simulink model "acoustic_delay_buffer"  (Simulink 9.2)
settings: Solver=FixedStepDiscrete  StartTime=0  StopTime=acoustic_delay_buffer_param.endTime  RelTol=1e-3  EnableMultiTasking=on
PreLoadFcn:
  | % Run the setup script when the model is opened
  | setup_acoustic_delay_buffer;
InitFcn:
  | % Run the setup script again just before the
  | % model is run, so that any updates made
  | % after opening are applied.
  | setup_acoustic_delay_buffer;
undefined symbols (not defined in the file or in its folder): acoustic_delay_buffer_param, AdvDSPBChannelOutDisplay, AdvDSPBDMemDisplay, AStInput, AStOutput, dpoly, dspba_ChannelInVis, dspba_ChannelOutVis, dspba_internal_get_channel_ports, DSPBAAvalonST, evalAionMaskParam, latency, primtype, UseDontCare, value
libraries: DSPBAPrim x45, simulink x4, DSPBABase x3, DSPBAModelBus x2
(part 1 of 2)
Description:
  | DSP Builder Advanced Template for Template Design implementing ModelIP designs
settings Model: LogicAnalyzerSignalOrdering=673dd956-a9b7-47c6-8e3b-b5370a165700,2ca13bd6-3b11-4a64-9ccb-860d4470aa9c,1314958b-2ca4-4760-b14e-21636fc16e8a,18024acf-8c31-4ed4-966b-9c5112f68f18,b16340d5-95cc-41ce-b9ba-3d9f2a82d5c7,73847741-1302-4618-ba98-6acef04c4683,30466ab8-321b-45d2-abc5-98b1f25c16af,0661e296-95ee-4d47-9664-915a724506db,a1263464-d66d-421f-b545-d698760bf497,336fe2d9-f44c-47a9-a8e5-5e40221b217f,f71103e9-4e69-4618-a9ca-5008dd724a19,a742d53d-581d-4b05-b348-192446bdeb24,b655c0ea-e5b7-4f9a-9095-04efa7391f59,5190fdba-c9e1-4656-be28-b079149338cb,ddf50ec1-edd7-49e5-a566-ac4f62c951d6,aaf5a439-c955-4ee6-b568-777acc1bd3bb,ac04c1fb-3b27-4459-9e9c-8231ad8ef4bf,6258e434-ad41-4b37-b0cd-7eb737f716c4,09754ba2-98e9-4803-bde8-10590804ee7c  Creator=mjervis  LastModifiedBy=trevorvannoy
settings Model: SuppressorTable=|
  | <?xml version="1.0" encoding="UTF-8" standalone="yes" ?>
  | <!DOCTYPE boost_serialization>
  | <boost_serialization signature="serialization::archive" version="15">
  | <DiagnosticSuppressor class_id="0" tracking_level="0" version="6">
  | 	<Table class_id="1" tracking_level="0" version="0">
  | 		<count>2</count>
  | 		<bucket_count>8</bucket_count>
  | 		<item_version>0</item_version>
  | 		<item class_id="2" tracking_level="0" version="0">
  | 			<first class_id="3" tracking_level="0" version="6">
  | 				<Source class_id="4" tracking_level="0" version="0">
  | 					<count>1</count>
  | 					<item_version>0</item_version>
  | 					<item>acoustic_delay_buffer/channel/LimitedCounter</item>
  | 				</Source>
  | 			</first>
  | 			<second class_id="5" tracking_level="0" version="6">
  | 				<SuppressedData class_id="6" tracking_level="0" version="0">
  | 					<count>2</count>
  | 					<bucket_count>8</bucket_count>
  | 					<item_version>0</item_version>
  | 					<item class_id="7" tracking_level="0" version="0">
  | 						<first class_id="8" tracking_level="0" version="6">
  | 							<ID>SimulinkFixedPoint:util:Overflowoccurred</ID>
  | 							<Cause>
  | 								<Source>
  | 									<count>0</count>
  | 									<item_version>0</item_version>
  | 								</Source>
  | 							</Cause>
  | 						</first>
  | 						<second class_id="9" tracking_level="0" version="6">
  | 							<Comment></Comment>
  | 							<User></User>
  | 							<LastModified class_id="10" tracking_level="0" version="0">
  | 								<ptime_date class_id="11" tracking_level="0" version="0">
  | 									<date>20160608</date>
  | 								</ptime_date>
  | 								<ptime_time_duration class_id="12" tracking_level="0" version="0">
  | 									<is_special>0</is_special>
  | 									<time_duration_hours>15</time_duration_hours>
  | 									<time_duration_minutes>23</time_duration_minutes>
  | 									<time_duration_seconds>17</time_duration_seconds>
  | 									<time_duration_fractional_seconds>0</time_duration_fractional_seconds>
  | 								</ptime_time_duration>
  | 							</LastModified>
  | 							<SuppressionType>1</SuppressionType>
  | 						</second>
  | 					</item>
  | 					<item>
  | 						<first>
  | 							<ID>Simulink:DataType:WarningOverFlowDetected</ID>
  | 							<Cause>
  | 								<Source>
  | 									<count>0</count>
  | 									<item_version>0</item_version>
  | 								</Source>
  | 							</Cause>
  | 						</first>
  | 						<second>
  | 							<Comment></Comment>
  | 							<User></User>
  | 							<LastModified>
  | 								<ptime_date>
  | 									<date>20160608</date>
  | 								</ptime_date>
  | 								<ptime_time_duration>
  | 									<is_special>0</is_special>
  | 									<time_duration_hours>15</time_duration_hours>
  | 									<time_duration_minutes>23</time_duration_minutes>
  | 									<time_duration_seconds>17</time_duration_seconds>
  | 									<time_duration_fractional_seconds>0</time_duration_fractional_seconds>
  | 								</ptime_time_duration>
  | 							</LastModified>
  | 							<SuppressionType>1</SuppressionType>
  | 						</second>
  | 					</item>
  | 				</SuppressedData>
  | 			</second>
  | 		</item>
  | 		<item>
  | 			<first>
  | 				<Source>
  | 					<count>1</count>
  | 					<item_version>0</item_version>
  | 					<item>acoustic_delay_buffer/adb/delay_write_en/LimitedCounter</item>
  | 				</Source>
  | 			</first>
  | 			<second>
  | 				<SuppressedData>
  | 					<count>2</count>
  | 					<bucket_count>8</bucket_count>
  | 					<item_version>0</item_version>
  | 					<item>
  | 						<first>
  | 							<ID>SimulinkFixedPoint:util:Overflowoccurred</ID>
  | 							<Cause>
  | 								<Source>
  | 									<count>0</count>
  | 									<item_version>0</item_version>
  | 								</Source>
  | 							</Cause>
  | 						</first>
  | 						<second>
  | 							<Comment></Comment>
  | 							<User></User>
  | 							<LastModified>
  | 								<ptime_date>
  | 									<date>20160608</date>
  | 								</ptime_date>
  | 								<ptime_time_duration>
  | 									<is_special>0</is_special>
  | 									<time_duration_hours>15</time_duration_hours>
  | 									<time_duration_minutes>23</time_duration_minutes>
  | 									<time_duration_seconds>17</time_duration_seconds>
  | 									<time_duration_fractional_seconds>0</time_duration_fractional_seconds>
  | 								</ptime_time_duration>
  | 							</LastModified>
  | 							<SuppressionType>1</SuppressionType>
  | 						</second>
  | 					</item>
  | 					<item>
  | 						<first>
  | 							<ID>Simulink:DataType:WarningOverFlowDetected</ID>
  | 							<Cause>
  | 								<Source>
  | 									<count>0</count>
  | 									<item_version>0</item_version>
  | 								</Source>
  | 							</Cause>
  | 						</first>
  | 						<second>
  | 							<Comment></Comment>
  | 							<User></User>
  | 							<LastModified>
  | 								<ptime_date>
  | 									<date>20160608</date>
  | 								</ptime_date>
  | 								<ptime_time_duration>
  | 									<is_special>0</is_special>
  | 									<time_duration_hours>15</time_duration_hours>
  | 									<time_duration_minutes>23</time_duration_minutes>
  | 									<time_duration_seconds>17</time_duration_seconds>
  | 									<time_duration_fractional_seconds>0</time_duration_fractional_seconds>
  | 								</ptime_time_duration>
  | 							</LastModified>
  | 							<SuppressionType>1</SuppressionType>
  | 						</second>
  | 					</item>
  | 				</SuppressedData>
  | 			</second>
  | 		</item>
  | 	</Table>
  | </DiagnosticSuppressor>
  | </boost_serialization>
settings Model: LogicAnalyzerGraphicalSettings=|
  | {
  |   "cursors" : {
  |     "activeCursor" : 0,
  |     "lockedCursors" : [
  | 
  |     ],
  |     "startingCursor" : 0,
  |     "times" : [
  |       1382
  |     ]
  |   },
  |   "global" : {
  |     "booleanDisplay" : "gradient",
  |     "color" : "#0073bd",
  |     "displayBusElementNames" : true,
  |     "displayShortNames" : true,
  |     "fontSize" : 12,
  |     "height" : 20,
  |     "recentlyUsedColors" : [
  |       "#7d2e8f",
  |       "#0073bd",
  |       "#0fffff",
  |       "default",
  |       "",
  |       "#ffff11",
  |       "#139fff"
  |     ]
  |   },
  |   "panels" : [
  |     {
  |       "height" : 100,
  |       "startingTrace" : 0,
  |       "traces" : [
  |         {
  |           "color" : "#ff6929",
  |           "height" : 30,
  |           "name" : "valid_stim",
  |           "signalId" : "18024acf-8c31-4ed4-966b-9c5112f68f18",
  |           "type" : "wave"
  |         },
  |         {
  |           "color" : "#ff6929",
  |           "height" : 30,
  |           "name" : "channel_stim",
  |           "signalId" : "b16340d5-95cc-41ce-b9ba-3d9f2a82d5c7",
  |           "type" : "wave"
  |         },
  |         {
  |           "color" : "#ff6929",
  |           "height" : 30,
  |           "name" : "data_stim",
  |           "signalId" : "73847741-1302-4618-ba98-6acef04c4683",
  |           "type" : "wave"
  |         },
  |         {
  |           "color" : "#0073bd",
  |           "height" : 30,
  |           "signalId" : "aaf5a439-c955-4ee6-b568-777acc1bd3bb",
  |           "type" : "wave"
  |         },
  |         {
  |           "color" : "#0073bd",
  |           "height" : 30,
  |           "signalId" : "ac04c1fb-3b27-4459-9e9c-8231ad8ef4bf",
  |           "type" : "wave"
  |         },
  |         {
  |           "color" : "#0073bd",
  |           "height" : 30,
  |           "signalId" : "ddf50ec1-edd7-49e5-a566-ac4f62c951d6",
  |           "type" : "wave"
  |         },
  |         {
  |           "color" : "#edb021",
  |           "height" : 30,
  |           "name" : "write_addr == delay",
  |           "signalId" : "1314958b-2ca4-4760-b14e-21636fc16e8a",
  |           "type" : "wave"
  |         },
  |         {
  |           "color" : "#edb021",
  |           "height" : 30,
  |           "name" : "valid_in",
  |           "signalId" : "a1263464-d66d-421f-b545-d698760bf497",
  |           "type" : "wave"
  |         },
  |         {
  |           "color" : "#b746ff",
  |           "height" : 30,
  |           "name" : "din",
  |           "signalId" : "336fe2d9-f44c-47a9-a8e5-5e40221b217f",
  |           "type" : "wave"
  |         },
  |         {
  |           "color" : "#b746ff",
  |           "height" : 30,
  |           "name" : "write",
  |           "signalId" : "a742d53d-581d-4b05-b348-192446bdeb24",
  |           "type" : "wave"
  |         },
  |         {
  |           "color" : "#b746ff",
  |           "height" : 30,
  |           "name" : "write_addr",
  |           "signalId" : "f71103e9-4e69-4618-a9ca-5008dd724a19",
  |           "type" : "wave"
  |         },
  |         {
  |           "color" : "#b746ff",
  |           "height" : 30,
  |           "name" : "read_addr",
  |           "signalId" : "b655c0ea-e5b7-4f9a-9095-04efa7391f59",
  |           "type" : "wave"
  |         },
  |         {
  |           "color" : "#b746ff",
  |           "height" : 30,
  |           "name" : "q1",
  |           "signalId" : "6258e434-ad41-4b37-b0cd-7eb737f716c4",
  |           "type" : "wave"
  |         },
  |         {
  |           "color" : "#b746ff",
  |           "height" : 30,
  |           "name" : "q2",
  |           "signalId" : "09754ba2-98e9-4803-bde8-10590804ee7c",
  |           "type" : "wave"
  |         },
  |         {
  |           "color" : "#78ab30",
  |           "height" : 30,
  |           "name" : "dout_buffer",
  |           "signalId" : "5190fdba-c9e1-4656-be28-b079149338cb",
  |           "type" : "wave"
  |         },
  |         {
  |           "color" : "#78ab30",
  |           "height" : 30,
  |           "name" : "ch_out_buffer",
  |           "signalId" : "30466ab8-321b-45d2-abc5-98b1f25c16af",
  |           "type" : "wave"
  |         },
  |         {
  |           "color" : "#78ab30",
  |           "height" : 30,
  |           "name" : "valid_out_buffer",
  |           "signalId" : "0661e296-95ee-4d47-9664-915a724506db",
  |           "type" : "wave"
  |         },
  |         {
  |           "color" : "#ff13a6",
  |           "height" : 30,
  |           "name" : "reset",
  |           "signalId" : "2ca13bd6-3b11-4a64-9ccb-860d4470aa9c",
  |           "type" : "wave"
  |         },
  |         {
  |           "color" : "#ff13a6",
  |           "height" : 30,
  |           "name" : "delay_comp",
  |           "signalId" : "673dd956-a9b7-47c6-8e3b-b5370a165700",
  |           "type" : "wave"
  |         }
  |       ],
  |       "yOffset" : 0
  |     }
  |   ],
  |   "timeAxis" : {
  |     "pixelsPerSecond" : 0.2014684101347109
  |   },
  |   "trigger" : {
  |     "enabled" : false,
  |     "mode" : "once",
  |     "samples" : 200,
  |     "signals" : {
  |     },
  |     "stages" : [
  |       {
  |         "conditions" : [
  | 
  |         ],
  |         "operator" : "AND"
  |       }
  |     ]
  |   }
  | }
settings DataIOCC: SignalLoggingSaveFormat=Dataset
settings OptimizationCC: BlockReduction=off  ConditionallyExecuteInputs=off  ExpressionDepthLimit=2147483647
settings DebuggingCC: SolverPrmCheckMsg=warning  InheritedTsInSrcMsg=none  MultiTaskRateTransMsg=warning  IntegerOverflowMsg=none  IntegerSaturationMsg=none

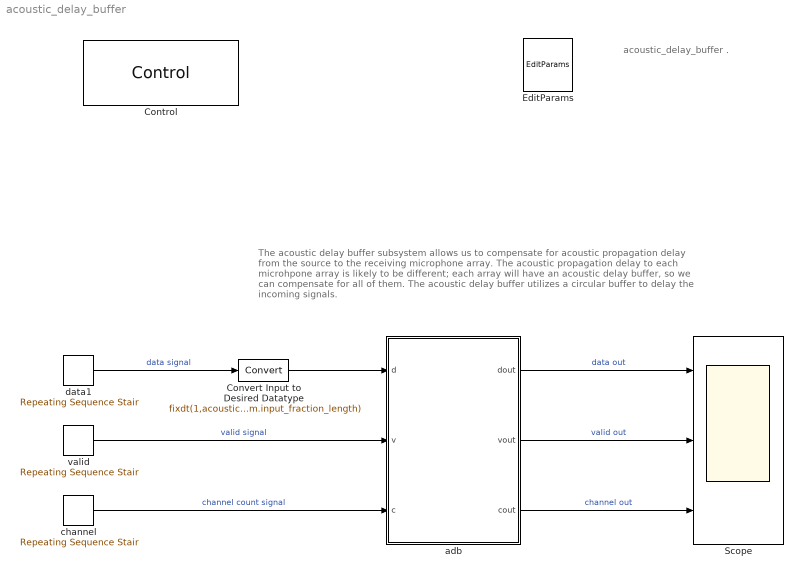
== system acoustic_delay_buffer ==
  note: The acoustic delay buffer subsystem allows us to compensate for acoustic propagation delay from the source to the receiving microphone array. The acoustic propagation delay to each microhpone array is likely to be different; each array will have an acoustic delay buffer, so we can compensate for all of them.
      |
      | The acoustic delay buffer utilizes a circular buffer to delay the incoming signals.
  note: acoustic_delay_buffer
      |                                          .
  Control : DSPBABase/Control  generate=on  language=VHDL  destination=./rtl  destination_gui=./rtl  make_full_path=off  quartus_work=../rtl  quartus_work_gui=../rtl  path_is_relative=on  autotestbench=off  signaldepth=2  coveragetestbench=off  logs=off  spacewidth=2  spacenum=1  addrwidth=10  datawidth=16  dataendian=Big Endian  hierarchicalnames=off  ramThresholdBits=-1  distRamThresholdBits=-1  mlabThresholdBits=-1  hardMultiplierThresholdLuts=-1  version=20090407  errorOnChanMismatch=on  errorOnGPIOMismatch=off  importModelsimResults=0  floatMismatchTolerance=-1.0  floatMismatchZeroTolerance=-1.0  cycleAccurate=off  reinterpretCastMult=off  paramFile=acoustic_delay_buffer_params.xml
  Convert Input to Desired Datatype : DataTypeConversion  OutDataTypeStr=fixdt(1,acoustic_delay_buffer_param.input_word_length,acoustic_delay_buffer_param.input_fraction_length)  SaturateOnIntegerOverflow=on
  EditParams : DSPBABase/EditParams  version=20090407
  Scope : Scope  NumInputPorts=3
  adb : Subsystem  TreatAsAtomicUnit=on
  channel : simulink/Sources/Repeating Sequence Stair  OutValues=acoustic_delay_buffer_param.chan_stim  tsamp=acoustic_delay_buffer_param.ClockCycle  OutMin=[]  OutMax=[]  OutDataTypeStr=uint8  OutputDataTypeScalingMode=uint8  OutDataType=uint8  ConRadixGroup=Best Precision: Vector-wise  OutScaling=2^-12
  data1 : simulink/Sources/Repeating Sequence Stair  OutValues=acoustic_delay_buffer_param.input_data  tsamp=acoustic_delay_buffer_param.ClockCycle  OutMin=[]  OutMax=[]  OutDataTypeStr=Inherit: Inherit via back propagation  OutDataType=fixdt('sfix16_En15')  ConRadixGroup=Best Precision: Vector-wise  OutScaling=[]
  valid : simulink/Sources/Repeating Sequence Stair  OutValues=[1, zeros(1, acoustic_delay_buffer_param.SampleTime-1)]  tsamp=acoustic_delay_buffer_param.ClockCycle  OutMin=[]  OutMax=[]  OutDataTypeStr=fixdt('boolean')  OutputDataTypeScalingMode=Specify via dialog  OutDataType=fixdt('boolean')  ConRadixGroup=Best Precision: Vector-wise  OutScaling=[]
  wires:
  valid/1 -> adb/2(v)  "valid signal"
  channel/1 -> adb/3(c)  "channel count signal"
  Convert Input to Desired Datatype/1 -> adb/1(d)
  data1/1 -> Convert Input to Desired Datatype/1  "data signal"
  adb/1(dout) -> Scope/1  "data out"
  adb/2(vout) -> Scope/2  "valid out"
  adb/3(cout) -> Scope/3  "channel out"

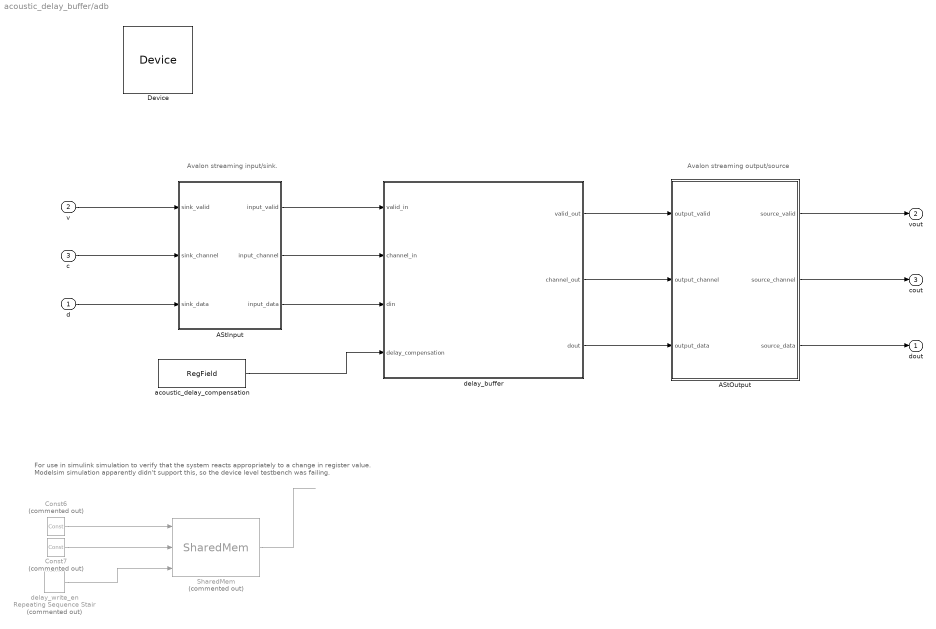
== system acoustic_delay_buffer/adb ==
  note: Avalon streaming input/sink.
  note: For use in simulink simulation to verify that the system reacts appropriately
      | to a change in register value. Modelsim simulation apparently didn't support this,
      | so the device level testbench was failing.
  note: Avalon streaming output/source
  d : Inport
  v : Inport  Port=2
  c : Inport  Port=3
  AStInput : Subsystem  AncestorBlock=DSPBAAvalonST/AStInput  InitFcn=warning('off','Simulink:Commands:LoadMdlParameterizedLink');  StopFcn=warning('on','Simulink:Commands:LoadMdlParameterizedLink');  mask(DSP Builder Advanced Blockset Avalon Streaming Input Interface){}
      mask help:
      | Avalon Streaming Input Interface
      |
      | Place this block at the front end of a system to generate the appropriate hw.tcl code for an Avalon Streaming interface with same name as the name of this block.
      mask Help: helpview(dspba.GetHelp('AStInput'));
      mask Display:
      | image('dspba_channel.jpg');
      | fprintf('Avalon-ST\nInput');
      | port_label('input',1,'sink_valid');
      | port_label('input',2,'sink_channel');
      | port_label('input',3,'sink_data');
      | port_label('output',1,'input_valid');
      | port_label('output',2,'input_channel');
      | port_label('output',3,'input_data');
  AStOutput : Subsystem  AncestorBlock=DSPBAAvalonST/AStOutput  InitFcn=warning('off','Simulink:Commands:LoadMdlParameterizedLink');  StopFcn=warning('on','Simulink:Commands:LoadMdlParameterizedLink');  mask(DSP Builder Advanced Blockset Avalon Streaming Output Interface){fifo_setup=[32 1 20]}
      mask prompts: fifo_setup "FIFO Setup [<_depth> <_fill_threshold> <_full_period>]:"
      mask help:
      | Avalon Streaming Output Interface
      |
      | Place this block the back end of a system to generate the appropriate hw.tcl code for an Avalon Streaming interface with same name as the name of this block.
      mask Help: helpview(dspba.GetHelp('AStOutput'));
      mask Display:
      | image('dspba_channel.jpg');
      | fprintf('Avalon-ST\nOutput');
      | port_label('input',1,'output_valid');
      | port_label('input',2,'output_channel');
      | port_label('input',3,'output_data');
      | port_label('output',1,'source_valid');
      | port_label('output',2,'source_channel');
      | port_label('output',3,'source_data');
  Const6 : DSPBAPrim/Const  Commented=on  primtype=const  nInputs=0  nOutputs=1  omode=Inherit via internal rule  otype=sfix(16)  scale=2^-15  rndmethod=Unbiased  factor=1  satmethod=Symmetric  shift_vec=[0 1 2 -1]  value=0  inPortNames=['+'; '+';]  outPortNames=[' ']  dspbaimage=dspba_prim.jpg  text=fprintf('%s', num2str(value));  style=Optimised  visibilities=8 + 1024  floatPrecision=float32_m23  version=20120820
  Const7 : DSPBAPrim/Const  Commented=on  primtype=const  nInputs=0  nOutputs=1  omode=Inherit via back propagation  otype=ufix(12)  scale=2^-15  rndmethod=Unbiased  factor=1  satmethod=Symmetric  shift_vec=[0 1 2 -1]  value=5  inPortNames=['+'; '+';]  outPortNames=[' ']  dspbaimage=dspba_prim.jpg  text=fprintf('%s', num2str(value));  style=Optimised  visibilities=8 + 1024  floatPrecision=float32_m23  version=20120820
  Device : DSPBABase/Device  family=Arria 10  deviceMember=Stratix IV GX  stratix4device=Stratix IV GX  hardcopy4device=HardCopy IV E  stratix5device=Stratix V GX  device=AUTO  speed=-2  stratixSpeed=-5  stratix2Speed=-3  stratix3Speed=-3  stratix4gxSpeed=-2  stratix4gtSpeed=-1  cyclone2Speed=-6  cyclone3Speed=-7  arria2Speed=-4  cyclone4eSpeed=-8  stratix5Speed=-3  arria5Speed=-4  arriaSpeed=-6  cyclone3lsSpeed=-7  cyclone5Speed=-6  arria2gzSpeed=-3  nightFurySpeed=-2  ecp2Speed=-7  hardcopycompat=off  version=20140217  max10flashmode=off  max10nomeminit=off
  SharedMem : DSPBAModelBus/SharedMem  Commented=on  mem_addr=0  mem_rwmode=Read/Write  mem_data=0  mem_init=on  mem_desc=Number of samples of delay to compensate for acoustic propagation delay  mem_mode=Specify via dialog  mem_type=ufix(acoustic_delay_buffer_param.addr_size)  mem_scale=1  SampleTime=-1  version=20090407
  acoustic_delay_compensation : DSPBAModelBus/RegField  reg_name=0  reg_rwmode=Read/Write  reg_msb=acoustic_delay_buffer_param.addr_size - 1  reg_lsb=0  reg_mode=Specify via dialog  reg_type=ufix(acoustic_delay_buffer_param.addr_size)  reg_scale=1  reg_init=0  reg_desc=Number of samples of delay to compensate for acoustic propagation delay  reg_modal=off  reg_desc0=0  reg_desc1=0  reg_desc2=0  reg_desc3=0  reg_desc4=0  reg_desc5=0  reg_desc6=0  reg_desc7=0  reg_addr=0  SampleTime=-1  version=20090407
  delay_buffer : Subsystem
  delay_write_en : simulink/Sources/Repeating Sequence Stair  Commented=on  OutValues=[zeros(1,acoustic_delay_buffer_param.endTime/4), 1, zeros(1, 3/4*acoustic_delay_buffer_param.endTime - 1)]  tsamp=acoustic_delay_buffer_param.ClockCycle  OutMin=[]  OutMax=[]  OutDataTypeStr=fixdt('boolean')  OutputDataTypeScalingMode=Specify via dialog  OutDataType=fixdt('boolean')  ConRadixGroup=Best Precision: Vector-wise  OutScaling=[]
  dout : Outport
  vout : Outport  Port=2
  cout : Outport  Port=3
  wires:
  SharedMem/1 -> ?
  delay_buffer/1(valid_out) -> AStOutput/1(output_valid)
  delay_buffer/2(channel_out) -> AStOutput/2(output_channel)
  delay_buffer/3(dout) -> AStOutput/3(output_data)
  AStInput/1(input_valid) -> delay_buffer/1(valid_in)
  AStInput/2(input_channel) -> delay_buffer/2(channel_in)
  AStInput/3(input_data) -> delay_buffer/3(din)
  delay_write_en/1 -> SharedMem/3
  v/1 -> AStInput/1(sink_valid)
  c/1 -> AStInput/2(sink_channel)
  d/1 -> AStInput/3(sink_data)
  AStOutput/2(source_channel) -> cout/1
  AStOutput/3(source_data) -> dout/1
  AStOutput/1(source_valid) -> vout/1
  Const7/1 -> SharedMem/2
  Const6/1 -> SharedMem/1
  acoustic_delay_compensation/1 -> delay_buffer/4(delay_compensation)

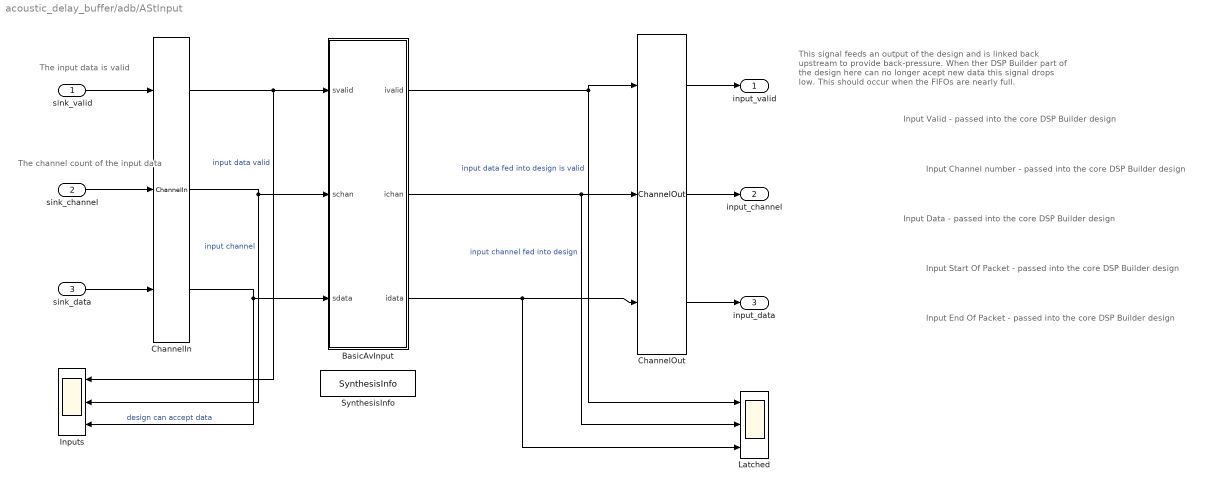
== system acoustic_delay_buffer/adb/AStInput ==
  note: Input End Of Packet - passed into the core DSP Builder design
  note: Input Start Of Packet - passed into the core DSP Builder design
  note: Input Data - passed into the core DSP Builder design
  note: Input Valid - passed into the core DSP Builder design
  note: This signal feeds an output of the design and is linked back
      | upstream to provide back-pressure. When ther DSP Builder
      | part of the design here can no longer acept new data this
      | signal drops low. This should occur when the FIFOs are nearly
      | full.
  note: Input Channel number - passed into the core DSP Builder design
  note: The channel count of the input data
  note: The input data is valid
  sink_valid : Inport  Tag=valid
      settings: AttributesFormatString=%<Tag>
  sink_channel : Inport  Tag=channel  Port=2
      settings: AttributesFormatString=%<Tag>
  sink_data : Inport  Tag=data  Port=3
      settings: AttributesFormatString=%<Tag>
  BasicAvInput : Subsystem
  ChannelIn : DSPBAPrim/ChannelIn  primtype=channelin  nInputs=dspba_internal_get_channel_ports(gcb)  nOutputs=dspba_internal_get_channel_ports(gcb)  omode=Inherit via internal rule  otype=sfix(16)  scale=2^-15  rndmethod=Unbiased  factor=1  satmethod=Symmetric  shift_vec=[0 1 2 -1]  value=1  inPortNames=['v'; 'c'; '0'; '1'; '2'; '3'; '4'; '5'; '6'; '7'; '8'; '9'; 'A'; 'B'; 'D'; 'E'; 'F'; 'G'; 'H'; 'I'; 'J'; 'K'; 'L'; 'M'; 'N'; 'O'; 'P'; 'Q'; 'R'; 'S'; 'T'; 'U'; 'W'; 'X'; 'Y'; 'Z']  outPortNames=['v'; 'c'; '0'; '1'; '2'; '3'; '4'; '5'; '6'; '7'; '8'; '9'; 'A'; 'B'; 'D'; 'E'; 'F'; 'G'; 'H'; 'I'; 'J'; 'K'; 'L'; 'M'; 'N'; 'O'; 'P'; 'Q'; 'R'; 'S'; 'T'; 'U'; 'W'; 'X'; 'Y'; 'Z']  dspbaimage=dspba_prim.jpg  text=fprintf('In');  style=Optimised  dataSignals=1  foldingEnabled=off  channels=1  sampleRate=200  packetBeginPresent=off  packetBeginEnabled=off  visibilities=dspba_ChannelInVis(gcb)  latencyCorrection=0  scheduleOrigin=on  version=20141013
  ChannelOut : DSPBAPrim/ChannelOut  primtype=channelout  nInputs=dspba_internal_get_channel_ports(gcb)  nOutputs=dspba_internal_get_channel_ports(gcb)  omode=Inherit via internal rule  otype=sfix(16)  scale=2^-15  rndmethod=Unbiased  factor=1  satmethod=Symmetric  shift_vec=[0 1 2 -1]  value=1  inPortNames=['v'; 'c'; '0'; '1'; '2'; '3'; '4'; '5'; '6'; '7'; '8'; '9'; 'A'; 'B'; 'D'; 'E'; 'F'; 'G'; 'H'; 'I'; 'J'; 'K'; 'L'; 'M'; 'N'; 'O'; 'P'; 'Q'; 'R'; 'S'; 'T'; 'U'; 'W'; 'X'; 'Y'; 'Z']  outPortNames=['v'; 'c'; '0'; '1'; '2'; '3'; '4'; '5'; '6'; '7'; '8'; '9'; 'A'; 'B'; 'D'; 'E'; 'F'; 'G'; 'H'; 'I'; 'J'; 'K'; 'L'; 'M'; 'N'; 'O'; 'P'; 'Q'; 'R'; 'S'; 'T'; 'U'; 'W'; 'X'; 'Y'; 'Z']  dspbaimage=dspba_prim.jpg  text=fprintf('Out%s', AdvDSPBChannelOutDisplay(latency));  style=Optimised  dataSignals=1  foldingEnabled=off  channels=1  sampleRate=200  packetBeginPresent=off  packetBeginEnabled=off  visibilities=dspba_ChannelOutVis(gcb)  latency=0  latencyCorrection=0  version=20141013
  Inputs : Scope  NumInputPorts=3
  Latched : Scope  NumInputPorts=3
  SynthesisInfo : DSPBAPrim/SynthesisInfo  primtype=synthinfo  nInputs=0  nOutputs=0  omode=Inherit via internal rule  otype=sfix(16)  scale=2^-15  rndmethod=Truncate  factor=1  satmethod=Symmetric  shift_vec=[0 1 2 -1]  value=99  inPortNames=[' '; ' ';]  outPortNames=[' ']  dspbaimage=dspba_prim_ctrl.jpg  text=fprintf('Style=%s', style);  style=Scheduled  visibilities=32768  constraintInUse=on  constraintRelation==  constraintLimit=0  bitAccurate=off  version=20150220
  input_valid : Outport  Tag=valid
      settings: AttributesFormatString=%<Tag>
  input_channel : Outport  Tag=channel  Port=2
      settings: AttributesFormatString=%<Tag>
  input_data : Outport  Tag=data  Port=3
      settings: AttributesFormatString=%<Tag>
  wires:
  ChannelOut/3 -> input_data/1
  BasicAvInput/1(ivalid) -> Latched/1, ChannelOut/1  "input data fed into design is valid"
  BasicAvInput/2(ichan) -> ChannelOut/2, Latched/2  "input channel fed into design"
  BasicAvInput/3(idata) -> Latched/3, ChannelOut/3
  ChannelIn/1 -> Inputs/1, BasicAvInput/1(svalid)  "input data valid"
  ChannelIn/2 -> Inputs/2, BasicAvInput/2(schan)  "input channel"
  ChannelIn/3 -> BasicAvInput/3(sdata), Inputs/3  "design can accept data"
  sink_valid/1 -> ChannelIn/1
  sink_channel/1 -> ChannelIn/2
  sink_data/1 -> ChannelIn/3
  ChannelOut/1 -> input_valid/1
  ChannelOut/2 -> input_channel/1

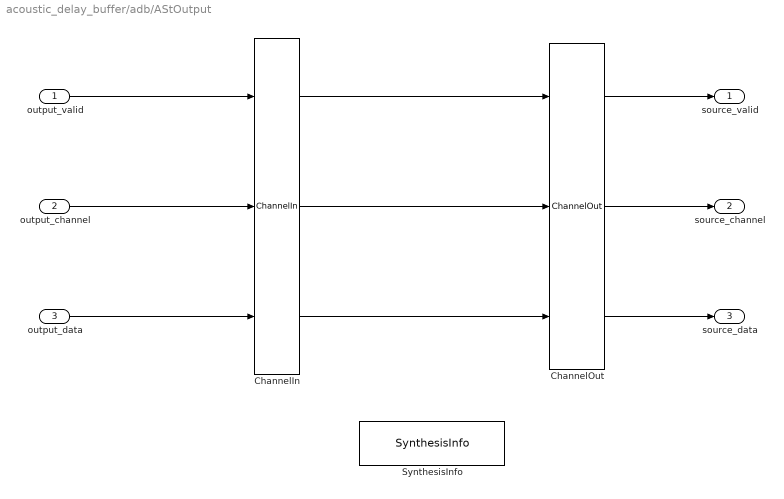
== system acoustic_delay_buffer/adb/AStOutput ==
  output_valid : Inport  Tag=valid
      settings: AttributesFormatString=%<Tag>
  output_channel : Inport  Tag=channel  Port=2
      settings: AttributesFormatString=%<Tag>
  output_data : Inport  Tag=data  Port=3
      settings: AttributesFormatString=%<Tag>
  ChannelIn : DSPBAPrim/ChannelIn  primtype=channelin  nInputs=dspba_internal_get_channel_ports(gcb)  nOutputs=dspba_internal_get_channel_ports(gcb)  omode=Inherit via internal rule  otype=sfix(16)  scale=2^-15  rndmethod=Unbiased  factor=1  satmethod=Symmetric  shift_vec=[0 1 2 -1]  value=1  inPortNames=['v'; 'c'; '0'; '1'; '2'; '3'; '4'; '5'; '6'; '7'; '8'; '9'; 'A'; 'B'; 'D'; 'E'; 'F'; 'G'; 'H'; 'I'; 'J'; 'K'; 'L'; 'M'; 'N'; 'O'; 'P'; 'Q'; 'R'; 'S'; 'T'; 'U'; 'W'; 'X'; 'Y'; 'Z']  outPortNames=['v'; 'c'; '0'; '1'; '2'; '3'; '4'; '5'; '6'; '7'; '8'; '9'; 'A'; 'B'; 'D'; 'E'; 'F'; 'G'; 'H'; 'I'; 'J'; 'K'; 'L'; 'M'; 'N'; 'O'; 'P'; 'Q'; 'R'; 'S'; 'T'; 'U'; 'W'; 'X'; 'Y'; 'Z']  dspbaimage=dspba_prim.jpg  text=fprintf('In');  style=Optimised  dataSignals=1  foldingEnabled=off  channels=1  sampleRate=200  packetBeginPresent=off  packetBeginEnabled=off  visibilities=dspba_ChannelInVis(gcb)  latencyCorrection=0  scheduleOrigin=on  version=20141013
  ChannelOut : DSPBAPrim/ChannelOut  primtype=channelout  nInputs=dspba_internal_get_channel_ports(gcb)  nOutputs=dspba_internal_get_channel_ports(gcb)  omode=Inherit via internal rule  otype=sfix(16)  scale=2^-15  rndmethod=Unbiased  factor=1  satmethod=Symmetric  shift_vec=[0 1 2 -1]  value=1  inPortNames=['v'; 'c'; '0'; '1'; '2'; '3'; '4'; '5'; '6'; '7'; '8'; '9'; 'A'; 'B'; 'D'; 'E'; 'F'; 'G'; 'H'; 'I'; 'J'; 'K'; 'L'; 'M'; 'N'; 'O'; 'P'; 'Q'; 'R'; 'S'; 'T'; 'U'; 'W'; 'X'; 'Y'; 'Z']  outPortNames=['v'; 'c'; '0'; '1'; '2'; '3'; '4'; '5'; '6'; '7'; '8'; '9'; 'A'; 'B'; 'D'; 'E'; 'F'; 'G'; 'H'; 'I'; 'J'; 'K'; 'L'; 'M'; 'N'; 'O'; 'P'; 'Q'; 'R'; 'S'; 'T'; 'U'; 'W'; 'X'; 'Y'; 'Z']  dspbaimage=dspba_prim.jpg  text=fprintf('Out%s', AdvDSPBChannelOutDisplay(latency));  style=Optimised  dataSignals=1  foldingEnabled=off  channels=1  sampleRate=200  packetBeginPresent=off  packetBeginEnabled=off  visibilities=dspba_ChannelOutVis(gcb)  latency=0  latencyCorrection=0  version=20141013
  SynthesisInfo : DSPBAPrim/SynthesisInfo  primtype=synthinfo  nInputs=0  nOutputs=0  omode=Inherit via internal rule  otype=sfix(16)  scale=2^-15  rndmethod=Truncate  factor=1  satmethod=Symmetric  shift_vec=[0 1 2 -1]  value=99  inPortNames=[' '; ' ';]  outPortNames=[' ']  dspbaimage=dspba_prim_ctrl.jpg  text=fprintf('Style=%s', style);  style=Scheduled  visibilities=32768  constraintInUse=on  constraintRelation==  constraintLimit=0  bitAccurate=off  version=20150220
  source_valid : Outport  Tag=valid
      settings: AttributesFormatString=%<Tag>
  source_channel : Outport  Tag=channel  Port=2
      settings: AttributesFormatString=%<Tag>
  source_data : Outport  Tag=data  Port=3
      settings: AttributesFormatString=%<Tag>
  wires:
  output_valid/1 -> ChannelIn/1
  output_channel/1 -> ChannelIn/2
  output_data/1 -> ChannelIn/3
  ChannelOut/1 -> source_valid/1
  ChannelOut/2 -> source_channel/1
  ChannelOut/3 -> source_data/1
  ChannelIn/1 -> ChannelOut/1
  ChannelIn/2 -> ChannelOut/2
  ChannelIn/3 -> ChannelOut/3

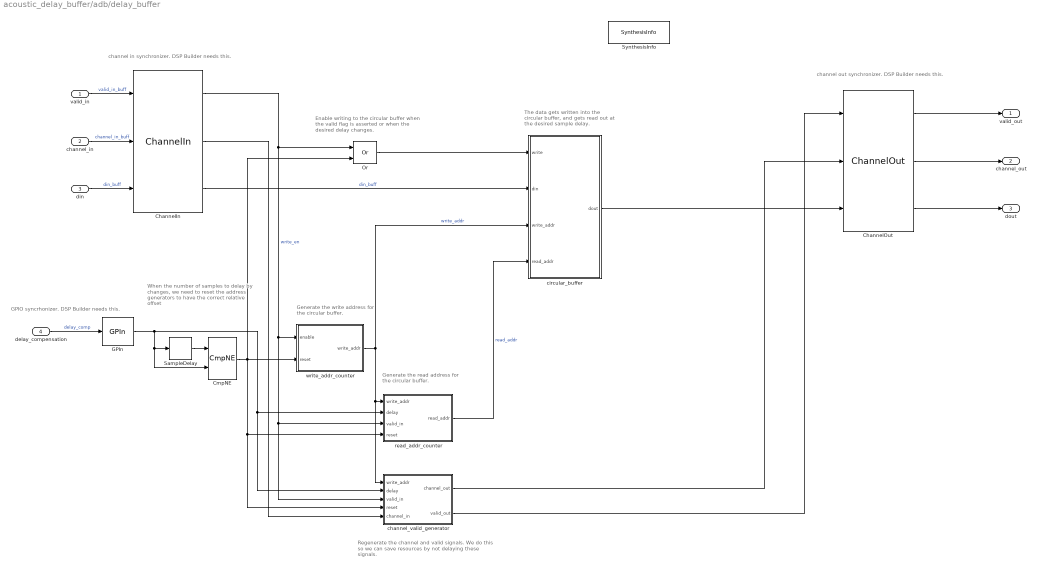
== system acoustic_delay_buffer/adb/delay_buffer ==
  note: Enable writing to the circular buffer when the valid flag is asserted or when the desired delay changes.
  note: The data gets written into the circular buffer, and gets read out at the desired sample delay.
  note: Regenerate the channel and valid signals. We do this so we can save resources by not delaying these signals.
  note: Generate the read address for the circular buffer.
  note: Generate the write address for the circular buffer.
  note: GPIO syncrhonizer. DSP Builder needs this.
  note: channel in synchronizer. DSP Builder needs this.
  note: When the number of samples to delay by changes,
      | we need to reset the address generators
      | to have the correct relative offset
  note: channel out synchronizer. DSP Builder needs this.
  valid_in : Inport
  channel_in : Inport  Port=2
  din : Inport  Port=3
  delay_compensation : Inport  Port=4
  ChannelIn : DSPBAPrim/ChannelIn  primtype=channelin  nInputs=dspba_internal_get_channel_ports(gcb)  nOutputs=dspba_internal_get_channel_ports(gcb)  omode=Inherit via internal rule  otype=sfix(16)  scale=2^-15  rndmethod=Unbiased  factor=1  satmethod=Symmetric  shift_vec=[0 1 2 -1]  value=1  inPortNames=['v'; 'c'; '0'; '1'; '2'; '3'; '4'; '5'; '6'; '7'; '8'; '9'; 'A'; 'B'; 'D'; 'E'; 'F'; 'G'; 'H'; 'I'; 'J'; 'K'; 'L'; 'M'; 'N'; 'O'; 'P'; 'Q'; 'R'; 'S'; 'T'; 'U'; 'W'; 'X'; 'Y'; 'Z']  outPortNames=['v'; 'c'; '0'; '1'; '2'; '3'; '4'; '5'; '6'; '7'; '8'; '9'; 'A'; 'B'; 'D'; 'E'; 'F'; 'G'; 'H'; 'I'; 'J'; 'K'; 'L'; 'M'; 'N'; 'O'; 'P'; 'Q'; 'R'; 'S'; 'T'; 'U'; 'W'; 'X'; 'Y'; 'Z']  dspbaimage=dspba_prim.jpg  text=fprintf('In');  style=Optimised  dataSignals=1  foldingEnabled=off  channels=1  sampleRate=200  packetBeginPresent=off  packetBeginEnabled=off  visibilities=dspba_ChannelInVis(gcb)  latencyCorrection=0  scheduleOrigin=on  version=20141013
  ChannelOut : DSPBAPrim/ChannelOut  primtype=channelout  nInputs=dspba_internal_get_channel_ports(gcb)  nOutputs=dspba_internal_get_channel_ports(gcb)  omode=Inherit via internal rule  otype=sfix(16)  scale=2^-15  rndmethod=Unbiased  factor=1  satmethod=Symmetric  shift_vec=[0 1 2 -1]  value=1  inPortNames=['v'; 'c'; '0'; '1'; '2'; '3'; '4'; '5'; '6'; '7'; '8'; '9'; 'A'; 'B'; 'D'; 'E'; 'F'; 'G'; 'H'; 'I'; 'J'; 'K'; 'L'; 'M'; 'N'; 'O'; 'P'; 'Q'; 'R'; 'S'; 'T'; 'U'; 'W'; 'X'; 'Y'; 'Z']  outPortNames=['v'; 'c'; '0'; '1'; '2'; '3'; '4'; '5'; '6'; '7'; '8'; '9'; 'A'; 'B'; 'D'; 'E'; 'F'; 'G'; 'H'; 'I'; 'J'; 'K'; 'L'; 'M'; 'N'; 'O'; 'P'; 'Q'; 'R'; 'S'; 'T'; 'U'; 'W'; 'X'; 'Y'; 'Z']  dspbaimage=dspba_prim.jpg  text=fprintf('Out%s', AdvDSPBChannelOutDisplay(latency));  style=Optimised  dataSignals=1  foldingEnabled=off  channels=1  sampleRate=200  packetBeginPresent=off  packetBeginEnabled=off  visibilities=dspba_ChannelOutVis(gcb)  latency=6  latencyCorrection=0  version=20141013
  CmpNE : DSPBAPrim/CmpNE  primtype=cmpne  nInputs=2  nOutputs=1  omode=boolean  otype=sfix(16)  scale=2^-15  rndmethod=Unbiased  factor=1  satmethod=Symmetric  shift_vec=[0 1 2 -1]  value=0  inPortNames=[' '; ' ';]  outPortNames=[' ']  dspbaimage=dspba_prim.jpg  text=fprintf('~=');  style=Optimised  visibilities=0  advOptions=[]  version=20130117
  GPIn : DSPBAPrim/GPIn  primtype=gpin  nInputs=evalAionMaskParam(gcb,'value',1)  nOutputs=evalAionMaskParam(gcb,'value',1)  omode=Inherit via internal rule  otype=sfix(16)  scale=2^-15  rndmethod=Unbiased  factor=1  satmethod=Symmetric  shift_vec=[0 1 2 -1]  value=1  inPortNames=[' ' ' ' ' ' ' ' ' ' ' ' ' ' ' ' ' ' ' ' ' ' ' ' ' ' ' ' ' ' ' ' ' ' ' ' ' ' ' ' ' ' ' ' ' ' ' ' ' ' ' ' ' ' ' ' ' ' ' ' ' ' ' ' ' ' ' ' ' ']'  outPortNames=[' ' ' ' ' ' ' ' ' ' ' ' ' ' ' ' ' ' ' ' ' ' ' ' ' ' ' ' ' ' ' ' ' ' ' ' ' ' ' ' ' ' ' ' ' ' ' ' ' ' ' ' ' ' ' ' ' ' ' ' ' ' ' ' ' ' ' ' ' ']'  dspbaimage=dspba_prim.jpg  text=fprintf('GPIn');  style=Optimised  visibilities=1024  latencyCorrection=0  scheduleOrigin=on  version=20090407
  Or : DSPBAPrim/Or  primtype=or  nInputs=2  nOutputs=1  omode=Inherit via internal rule  otype=sfix(16)  scale=2^-15  rndmethod=Unbiased  factor=1  satmethod=Symmetric  shift_vec=[0 1 2 -1]  value=0  inPortNames=[' '; ' '; ' '; ' '; ' '; ' '; ' '; ' '; ' '; ' '; ' '; ' '; ' '; ' '; ' '; ' '; ]  outPortNames=[' ']  dspbaimage=dspba_prim.jpg  text=fprintf('|');  style=Optimised  visibilities=8+2  version=20090407
  SampleDelay : DSPBAPrim/SampleDelay  primtype=sampdelay  nInputs=1  nOutputs=1  omode=Inherit via internal rule  otype=sfix(16)  scale=2^-15  rndmethod=Unbiased  factor=1  satmethod=Symmetric  shift_vec=[0 1 2 -1]  value=1  inPortNames=[' '; ' ';]  outPortNames=[' ']  dspbaimage=dspba_prim.jpg  text=dpoly(1, eye(1,value+1), 'z')  style=Optimised  visibilities=8 + 1024 + 2^17 + 2^18  flexible=off  slackgroup=0  augmented=0  version=20090407  advOptions=[]
  SynthesisInfo : DSPBAPrim/SynthesisInfo  primtype=synthinfo  nInputs=0  nOutputs=0  omode=Inherit via internal rule  otype=sfix(16)  scale=2^-15  rndmethod=Truncate  factor=1  satmethod=Symmetric  shift_vec=[0 1 2 -1]  value=99  inPortNames=[' '; ' ';]  outPortNames=[' ']  dspbaimage=dspba_prim_ctrl.jpg  text=fprintf('Style=%s', style);  style=Scheduled  visibilities=2^17+2^18+2^19+2^20  constraintInUse=off  constraintRelation=>  constraintLimit=2  bitAccurate=off  version=20150220
  channel_valid_generator : Subsystem
  circular_buffer : Subsystem
  read_addr_counter : Subsystem
  write_addr_counter : Subsystem
  valid_out : Outport
  channel_out : Outport  Port=2
  dout : Outport  Port=3
  wires:
  din/1 -> ChannelIn/3  "din_buff"
  channel_in/1 -> ChannelIn/2  "channel_in_buff"
  valid_in/1 -> ChannelIn/1  "valid_in_buff"
  write_addr_counter/1(write_addr) -> read_addr_counter/1(write_addr), channel_valid_generator/1(write_addr), circular_buffer/3(write_addr)  "write_addr"
  delay_compensation/1 -> GPIn/1  "delay_comp"
  ChannelIn/3 -> circular_buffer/2(din)  "din_buff"
  read_addr_counter/1(read_addr) -> circular_buffer/4(read_addr)  "read_addr"
  circular_buffer/1(dout) -> ChannelOut/3
  ChannelIn/1 -> channel_valid_generator/3(valid_in), read_addr_counter/3(valid_in), write_addr_counter/1(enable), Or/1  "write_en"
  channel_valid_generator/1(channel_out) -> ChannelOut/2
  channel_valid_generator/2(valid_out) -> ChannelOut/1
  ChannelOut/1 -> valid_out/1
  ChannelOut/2 -> channel_out/1
  ChannelOut/3 -> dout/1
  ChannelIn/2 -> channel_valid_generator/5(channel_in)
  SampleDelay/1 -> CmpNE/1
  GPIn/1 -> channel_valid_generator/2(delay), read_addr_counter/2(delay), CmpNE/2, SampleDelay/1
  CmpNE/1 -> Or/2, channel_valid_generator/4(reset), read_addr_counter/4(reset), write_addr_counter/2(reset)
  Or/1 -> circular_buffer/1(write)

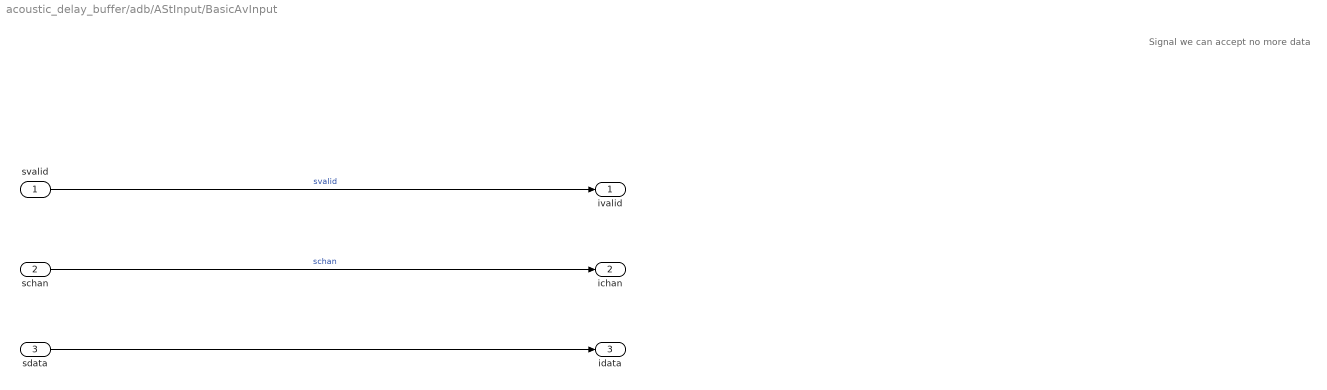
== system acoustic_delay_buffer/adb/AStInput/BasicAvInput ==
  note: Signal we can accept no more data
  svalid : Inport
  schan : Inport  Port=2
  sdata : Inport  Port=3
  ivalid : Outport
  ichan : Outport  Port=2
  idata : Outport  Port=3
  wires:
  svalid/1 -> ivalid/1  "svalid"
  sdata/1 -> idata/1
  schan/1 -> ichan/1  "schan"

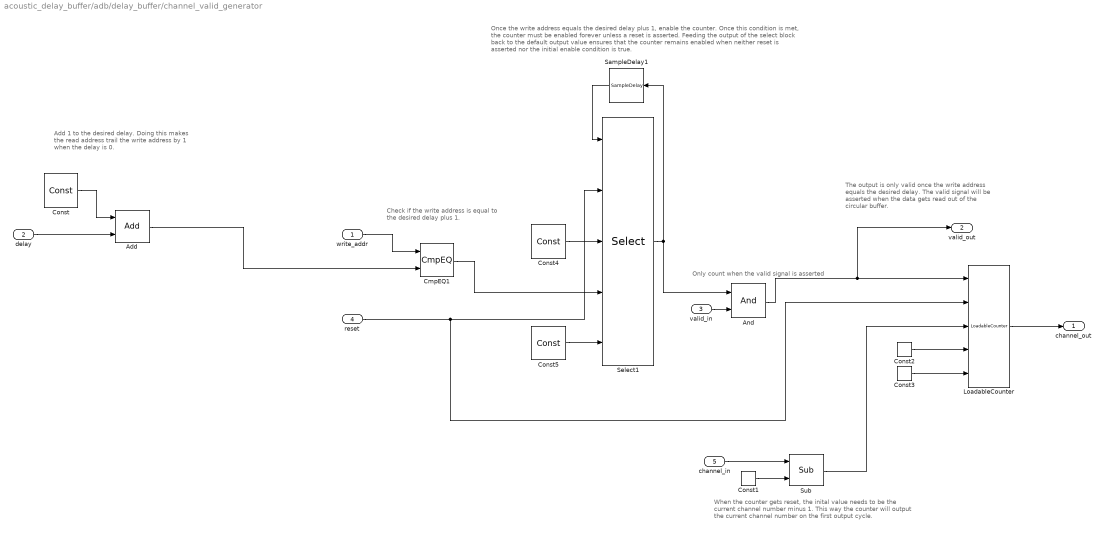
== system acoustic_delay_buffer/adb/delay_buffer/channel_valid_generator ==
  note: When the counter gets reset, the inital value needs to be the current channel number minus 1. This way the counter will output the current channel number on the first output cycle.
  note: The output is only valid once the write address equals the desired delay. The valid signal will be asserted when the data gets read out of the circular buffer.
  note: Add 1 to the desired delay. Doing this makes the read address trail the write address by 1 when the delay is 0.
  note: Only count when the valid signal is asserted
  note: Once the write address equals the desired delay plus 1, enable the counter. Once this condition is met, the counter must be enabled forever unless a reset is asserted. Feeding the output of the select block back to the default output value ensures that the counter remains enabled when neither reset is asserted nor the initial enable condition is true.
  note: Check if the write address is equal to the desired delay plus 1.
  write_addr : Inport
  delay : Inport  Port=2
  valid_in : Inport  Port=3
  reset : Inport  Port=4
  channel_in : Inport  Port=5
  Add : DSPBAPrim/Add  primtype=add  nInputs=evalAionMaskParam(gcb,'value',1)  nOutputs=1  omode=Inherit via internal rule with word growth  otype=sfix(16)  scale=2^-15  rndmethod=Unbiased  factor=1  satmethod=Symmetric  shift_vec=[0 1 2 -1]  value=2  inPortNames=[' '; ' ';]  outPortNames=[' ']  dspbaimage=dspba_prim.jpg  text=fprintf('+');  style=Optimised  visibilities=1032+2^17+2^18+2^19  genFPC=off  floatRounding=correct  advOptions=[]  version=20130821
  And : DSPBAPrim/And  primtype=and  nInputs=2  nOutputs=1  omode=Inherit via internal rule  otype=sfix(16)  scale=2^-15  rndmethod=Unbiased  factor=1  satmethod=Symmetric  shift_vec=[0 1 2 -1]  value=0  inPortNames=[' '; ' '; ' '; ' '; ' '; ' '; ' '; ' '; ' '; ' '; ' '; ' '; ' '; ' '; ' '; ' '; ]  outPortNames=[' ']  dspbaimage=dspba_prim.jpg  text=fprintf('&');  style=Optimised  visibilities=8+2  version=20090407
  CmpEQ1 : DSPBAPrim/CmpEQ  primtype=cmpeq  nInputs=2  nOutputs=1  omode=boolean  otype=sfix(16)  scale=2^-15  rndmethod=Unbiased  factor=1  satmethod=Symmetric  shift_vec=[0 1 2 -1]  value=0  inPortNames=[' '; ' ';]  outPortNames=[' ']  dspbaimage=dspba_prim.jpg  text=fprintf('==');  style=Optimised  visibilities=0  advOptions=[]  version=20130117
  Const : DSPBAPrim/Const  primtype=const  nInputs=0  nOutputs=1  omode=Inherit via internal rule  otype=sfix(16)  scale=2^-15  rndmethod=Unbiased  factor=1  satmethod=Symmetric  shift_vec=[0 1 2 -1]  value=1  inPortNames=['+'; '+';]  outPortNames=[' ']  dspbaimage=dspba_prim.jpg  text=fprintf('%s', num2str(value));  style=Optimised  visibilities=8 + 1024  floatPrecision=float32_m23  version=20120820
  Const1 : DSPBAPrim/Const  primtype=const  nInputs=0  nOutputs=1  omode=Specify via dialog  otype=uint(8)  scale=1  rndmethod=Unbiased  factor=1  satmethod=Symmetric  shift_vec=[0 1 2 -1]  value=1  inPortNames=['+'; '+';]  outPortNames=[' ']  dspbaimage=dspba_prim.jpg  text=fprintf('%s', num2str(value));  style=Optimised  visibilities=8 + 1024  floatPrecision=float32_m23  version=20120820
  Const2 : DSPBAPrim/Const  primtype=const  nInputs=0  nOutputs=1  omode=Inherit via internal rule  otype=sfix(16)  scale=2^-15  rndmethod=Unbiased  factor=1  satmethod=Symmetric  shift_vec=[0 1 2 -1]  value=1  inPortNames=['+'; '+';]  outPortNames=[' ']  dspbaimage=dspba_prim.jpg  text=fprintf('%s', num2str(value));  style=Optimised  visibilities=8 + 1024  floatPrecision=float32_m23  version=20120820
  Const3 : DSPBAPrim/Const  primtype=const  nInputs=0  nOutputs=1  omode=Inherit via internal rule  otype=sfix(16)  scale=2^-15  rndmethod=Unbiased  factor=1  satmethod=Symmetric  shift_vec=[0 1 2 -1]  value=acoustic_delay_buffer_param.ChanCount  inPortNames=['+'; '+';]  outPortNames=[' ']  dspbaimage=dspba_prim.jpg  text=fprintf('%s', num2str(value));  style=Optimised  visibilities=8 + 1024  floatPrecision=float32_m23  version=20120820
  Const4 : DSPBAPrim/Const  primtype=const  nInputs=0  nOutputs=1  omode=Inherit via internal rule  otype=sfix(16)  scale=2^-15  rndmethod=Unbiased  factor=1  satmethod=Symmetric  shift_vec=[0 1 2 -1]  value=0  inPortNames=['+'; '+';]  outPortNames=[' ']  dspbaimage=dspba_prim.jpg  text=fprintf('%s', num2str(value));  style=Optimised  visibilities=8 + 1024  floatPrecision=float32_m23  version=20120820
  Const5 : DSPBAPrim/Const  primtype=const  nInputs=0  nOutputs=1  omode=Inherit via internal rule  otype=sfix(16)  scale=2^-15  rndmethod=Unbiased  factor=1  satmethod=Symmetric  shift_vec=[0 1 2 -1]  value=1  inPortNames=['+'; '+';]  outPortNames=[' ']  dspbaimage=dspba_prim.jpg  text=fprintf('%s', num2str(value));  style=Optimised  visibilities=8 + 1024  floatPrecision=float32_m23  version=20120820
  LoadableCounter : DSPBAPrim/LoadableCounter  primtype=loadablecounter  nInputs=5  nOutputs=1  omode=Specify via dialog  otype=ufix(8)  scale=2^-0  rndmethod=Unbiased  factor=1  satmethod=Symmetric  shift_vec=[0 1 2 -1]  value=[acoustic_delay_buffer_param.ChanCount - 1 acoustic_delay_buffer_param.ChanCount 1]  inPortNames=['en';'ld';'i ';'s ';'m ']  outPortNames=[' ']  dspbaimage=dspba_prim.jpg  text=fprintf('loadable\ncounter\n[%d %d %d]', value(1), value(2), value(3));  style=Optimised  visibilities=8 + 1024  version=20090407
  SampleDelay1 : DSPBAPrim/SampleDelay  primtype=sampdelay  nInputs=1  nOutputs=1  omode=Inherit via internal rule  otype=sfix(16)  scale=2^-15  rndmethod=Unbiased  factor=1  satmethod=Symmetric  shift_vec=[0 1 2 -1]  value=1  inPortNames=[' '; ' ';]  outPortNames=[' ']  dspbaimage=dspba_prim.jpg  text=dpoly(1, eye(1,value+1), 'z')  style=Optimised  visibilities=8 + 1024 + 2^17 + 2^18  flexible=off  slackgroup=0  augmented=0  version=20090407  advOptions=[]
  Select1 : DSPBAPrim/Select  primtype=select  nInputs=str2num(get_param(gcb,'value'))*2+1  nOutputs=1  omode=boolean  otype=sfix(16)  scale=2^-15  rndmethod=Unbiased  factor=1  satmethod=Symmetric  shift_vec=[0 1 2 -1]  value=2  inPortNames=['d'; '0'; 'a'; '1'; 'b'; '2'; 'c'; '3'; 'd'; '4'; 'e'; '5'; 'f'; '6'; 'g'; '7'; 'h'; '8'; 'i'; '9'; 'j']  outPortNames=[' ']  dspbaimage=dspba_prim.jpg  text=fprintf('%s', primtype);  style=Optimised  visibilities=8 + 1024  version=20090407
  Sub : DSPBAPrim/Sub  primtype=sub  nInputs=2  nOutputs=1  omode=Inherit via internal rule  otype=sfix(16)  scale=2^-15  rndmethod=Unbiased  factor=1  satmethod=Symmetric  shift_vec=[0 1 2 -1]  value=0  inPortNames=['+'; '-';]  outPortNames=[' ']  dspbaimage=dspba_prim.jpg  text=fprintf('-');  style=Optimised  visibilities=8+2^17+2^18  floatRounding=correct  advOptions=[]  version=20130115
  channel_out : Outport
  valid_out : Outport  Port=2
  wires:
  And/1 -> LoadableCounter/1, valid_out/1
  LoadableCounter/1 -> channel_out/1
  reset/1 -> LoadableCounter/2, Select1/2
  Const3/1 -> LoadableCounter/5
  Const2/1 -> LoadableCounter/4
  Const4/1 -> Select1/3
  SampleDelay1/1 -> Select1/1
  write_addr/1 -> CmpEQ1/1
  valid_in/1 -> And/2
  Select1/1 -> And/1, SampleDelay1/1
  Const5/1 -> Select1/5
  CmpEQ1/1 -> Select1/4
  Const/1 -> Add/1
  Add/1 -> CmpEQ1/2
  delay/1 -> Add/2
  channel_in/1 -> Sub/1
  Const1/1 -> Sub/2
  Sub/1 -> LoadableCounter/3

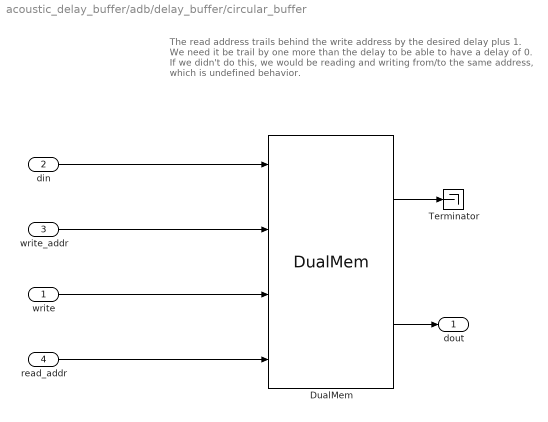
== system acoustic_delay_buffer/adb/delay_buffer/circular_buffer ==
  note: The read address trails behind the write address by the desired delay plus 1. We need it be trail by one more than the delay to be able to have a delay of 0. If we didn't do this, we would be reading and writing from/to the same address, which is undefined behavior.
  write : Inport
  din : Inport  Port=2
  write_addr : Inport  Port=3
  read_addr : Inport  Port=4
  DualMem : DSPBAPrim/DualMem  primtype=dualmem  nInputs=4  nOutputs=2  omode=Inherit via internal rule  otype=sfix(16)  scale=2^-15  rndmethod=Unbiased  factor=1  satmethod=Symmetric  shift_vec=[0 1 2 -1]  value=[zeros(acoustic_delay_buffer_param.buffer_size, 1)]  inPortNames=['d1'; 'a1'; 'w1'; 'a2']  outPortNames=['q1'; 'q2']  dspbaimage=dspba_prim.jpg  text=fprintf('dmem%s',AdvDSPBDMemDisplay(UseDontCare));  style=Optimised  visibilities=8 + 1024 + 2^17 + 2^18  UseDontCare=on  TwinWritePorts=off  version=20141001
  Terminator : Terminator
  dout : Outport
  wires:
  DualMem/2 -> dout/1
  write_addr/1 -> DualMem/2
  read_addr/1 -> DualMem/4
  DualMem/1 -> Terminator/1
  write/1 -> DualMem/3
  din/1 -> DualMem/1
